simulink model "Ju_FCM_v2_03252019_Arash"  (R2018a)
settings: Solver=VariableStepAuto  StartTime=0.0  StopTime=.5  MaxStep=1e-6  RelTol=1e-3
values from neighbouring files (symbols this model uses):
  C_FCM = 100e-6    (= 0.0001)    [Ju_parameters_FCM_v2_03252019_Arash.m]
  f = 50    [Ju_parameters_FCM_v2_03252019_Arash.m]
  L = XL/(2*pi*f)    [Ju_parameters_FCM_v2_03252019_Arash.m]
  n = 4    [Ju_parameters_FCM_v2_03252019_Arash.m]
  R = Z*pf    (= 20)    [Ju_parameters_FCM_v2_03252019_Arash.m]
libraries: powerlib x21, powerlib_meascontrol x4
settings Model: Creator=JHK5183  LastModifiedBy=kzs1012
settings SolverCC: ZeroCrossAlgorithm=Adaptive
settings DebuggingCC: MaxConsecutiveZCsMsg=none

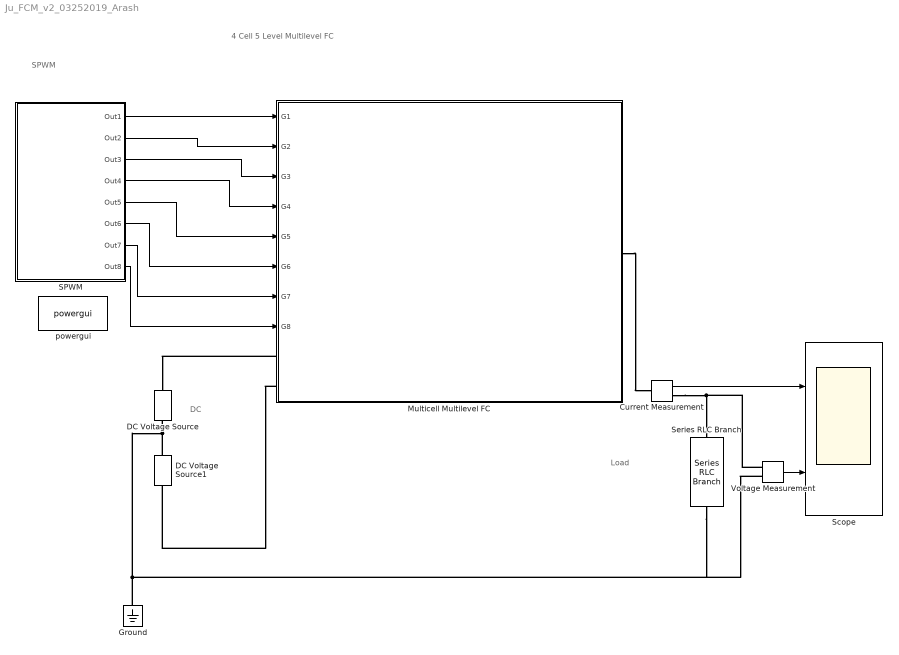
== system Ju_FCM_v2_03252019_Arash ==
  note: Load
  note: DC
  note: 4 Cell 5 Level Multilevel FC
  note: SPWM
  Current Measurement : powerlib/Measurements/Current Measurement  PhasorSimulation=off  OutputType=Complex  PSBequivalent=0
  DC Voltage Source : powerlib/Electrical Sources/DC Voltage Source  Amplitude=E/2  Measurements=None
  DC Voltage Source1 : powerlib/Electrical Sources/DC Voltage Source  Amplitude=E/2  Measurements=None
  Ground : powerlib/Elements/Ground  LConnTagsString=a
  Multicell Multilevel FC : Subsystem
  SPWM : Subsystem
  Scope : Scope  NumInputPorts=2
  Series RLC Branch : powerlib/Elements/Series RLC Branch  LConnTagsString=__new0  RConnTagsString=__new0  BranchType=RL  Resistance=R  Inductance=L  SetiL0=off  InitialCurrent=0  Capacitance=1e-6  Setx0=off  InitialVoltage=0  Measurements=None
  Voltage Measurement : powerlib/Measurements/Voltage Measurement  PhasorSimulation=off  OutputType=Complex  PSBequivalent=0
  powergui : powerlib/powergui  Priority=1  SimulationMode=Continuous  SampleTime=50e-6  frequency=60  Iterations=50  frequencyindice=0  Pbase=100e6  ErrMax=1e-4  UnitsV=kV  UnitsW=MW  buscounter=0  FunctionMessages=off  echomessages=off  EnableUseOfTLC=off  CurrentSourceSwitches=off  DisableSnubberDevices=off  DisableRonSwitches=off  DisableVfSwitches=off  DisplayEquations=off  SolverType=Tustin/Backward Euler (TBE)  Interpol=off  ExternalGateDelay=off  methode=off  Ts=100  x0status=blocks  SPID=on  SwTol=0  HookPort=off  RestoreLinks=warning  ResistiveCurrentMeasurement=off  Frange=[0:2:500]  Ylog=off  Xlog=on  ShowGrid=off  save=off  variable=ZData  structure=0  ZoomFFT=off  StartTime=0.0  cycles=1  DisplayStyle=1  fundamental=60  FreqAxis=off  MaxFrequency=1000  frequencyindicesteady=1  RmsSteady=1  display=off
  wires:
  Current Measurement/1 -> Scope/1
  Voltage Measurement/1 -> Scope/2
  SPWM/1(Out1) -> Multicell Multilevel FC/1(G1)
  SPWM/2(Out2) -> Multicell Multilevel FC/2(G2)
  SPWM/3(Out3) -> Multicell Multilevel FC/3(G3)
  SPWM/4(Out4) -> Multicell Multilevel FC/4(G4)
  SPWM/5(Out5) -> Multicell Multilevel FC/5(G5)
  SPWM/6(Out6) -> Multicell Multilevel FC/6(G6)
  SPWM/7(Out7) -> Multicell Multilevel FC/7(G7)
  SPWM/8(Out8) -> Multicell Multilevel FC/8(G8)
  connections:
  Multicell Multilevel FC/LConn1 -- DC Voltage Source/RConn1
  Voltage Measurement/LConn1 -- Current Measurement/RConn1 -- Series RLC Branch/LConn1
  DC Voltage Source/LConn1 -- Series RLC Branch/RConn1 -- Voltage Measurement/LConn2 -- Ground/LConn1 -- DC Voltage Source1/RConn1
  Multicell Multilevel FC/LConn2 -- DC Voltage Source1/LConn1
  Multicell Multilevel FC/RConn1 -- Current Measurement/LConn1

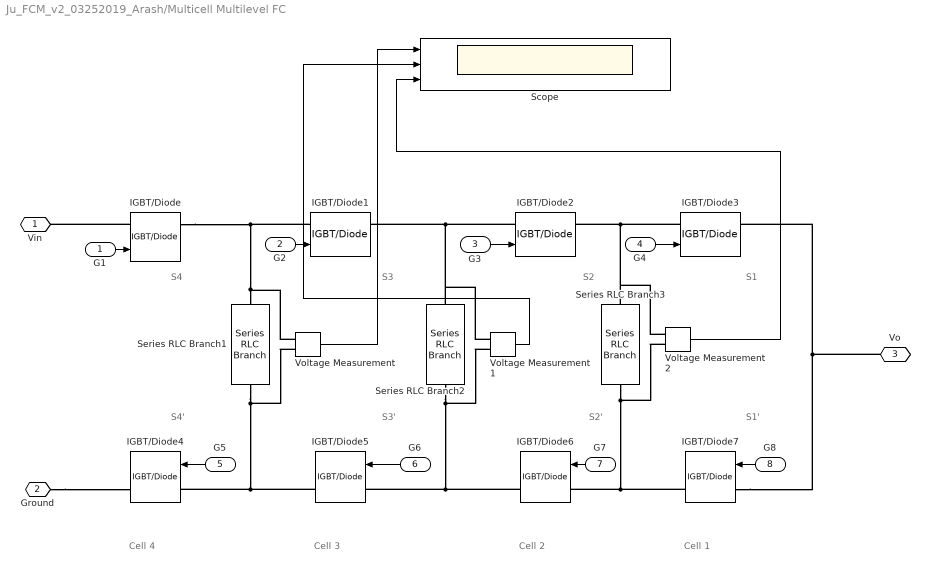
== system Ju_FCM_v2_03252019_Arash/Multicell Multilevel FC ==
  note: Cell 4
  note: S4
  note: S3
  note: S2
  note: S1
  note: S4'
  note: S3'
  note: S2'
  note: S1'
  note: Cell 3
  note: Cell 2
  note: Cell 1
  G1 : Inport
  G2 : Inport  Port=2
  G3 : Inport  Port=3
  G4 : Inport  Port=4
  G5 : Inport  Port=5
  G6 : Inport  Port=6
  G7 : Inport  Port=7
  G8 : Inport  Port=8
  IGBT/Diode{,1..7} (8 alike) : powerlib/Power Electronics/IGBT//Diode  Ron=1e-3  Rs=1e5  Cs=inf  Measurements=on
  Scope : Scope  NumInputPorts=3
  Series RLC Branch1 : powerlib/Elements/Series RLC Branch  LConnTagsString=__new0  RConnTagsString=__new0  BranchType=C  Resistance=1  Inductance=1e-3  SetiL0=off  InitialCurrent=0  Capacitance=C_FCM  Setx0=on  InitialVoltage=0  Measurements=None
  Series RLC Branch2 : powerlib/Elements/Series RLC Branch  LConnTagsString=__new0  RConnTagsString=__new0  BranchType=C  Resistance=1  Inductance=1e-3  SetiL0=off  InitialCurrent=0  Capacitance=C_FCM  Setx0=on  InitialVoltage=0  Measurements=None
  Series RLC Branch3 : powerlib/Elements/Series RLC Branch  LConnTagsString=__new0  RConnTagsString=__new0  BranchType=C  Resistance=1  Inductance=1e-3  SetiL0=off  InitialCurrent=0  Capacitance=C_FCM  Setx0=on  InitialVoltage=0  Measurements=None
  Voltage Measurement : powerlib/Measurements/Voltage Measurement  PhasorSimulation=off  OutputType=Complex  PSBequivalent=0
  Voltage Measurement1 : powerlib/Measurements/Voltage Measurement  PhasorSimulation=off  OutputType=Complex  PSBequivalent=0
  Voltage Measurement2 : powerlib/Measurements/Voltage Measurement  PhasorSimulation=off  OutputType=Complex  PSBequivalent=0
  Vin : PMIOPort  Side=Left
  Ground : PMIOPort  Port=2  Side=Left
  Vo : PMIOPort  Port=3  Side=Right
  wires:
  G1/1 -> IGBT/Diode/1
  G6/1 -> IGBT/Diode5/1
  G2/1 -> IGBT/Diode1/1
  G3/1 -> IGBT/Diode2/1
  G4/1 -> IGBT/Diode3/1
  G5/1 -> IGBT/Diode4/1
  G7/1 -> IGBT/Diode6/1
  G8/1 -> IGBT/Diode7/1
  Voltage Measurement/1 -> Scope/1
  Voltage Measurement1/1 -> Scope/2
  Voltage Measurement2/1 -> Scope/3
  connections:
  IGBT/Diode7/LConn1 -- IGBT/Diode3/RConn1 -- Vo/RConn1
  IGBT/Diode/RConn1 -- IGBT/Diode1/LConn1 -- Voltage Measurement/LConn1 -- Series RLC Branch1/LConn1
  IGBT/Diode/LConn1 -- Vin/RConn1
  IGBT/Diode2/LConn1 -- Voltage Measurement1/LConn1 -- Series RLC Branch2/LConn1 -- IGBT/Diode1/RConn1
  IGBT/Diode3/LConn1 -- Voltage Measurement2/LConn1 -- Series RLC Branch3/LConn1 -- IGBT/Diode2/RConn1
  Ground/RConn1 -- IGBT/Diode4/RConn1
  Series RLC Branch1/RConn1 -- Voltage Measurement/LConn2 -- IGBT/Diode4/LConn1 -- IGBT/Diode5/RConn1
  Series RLC Branch2/RConn1 -- Voltage Measurement1/LConn2 -- IGBT/Diode5/LConn1 -- IGBT/Diode6/RConn1
  Series RLC Branch3/RConn1 -- Voltage Measurement2/LConn2 -- IGBT/Diode6/LConn1 -- IGBT/Diode7/RConn1

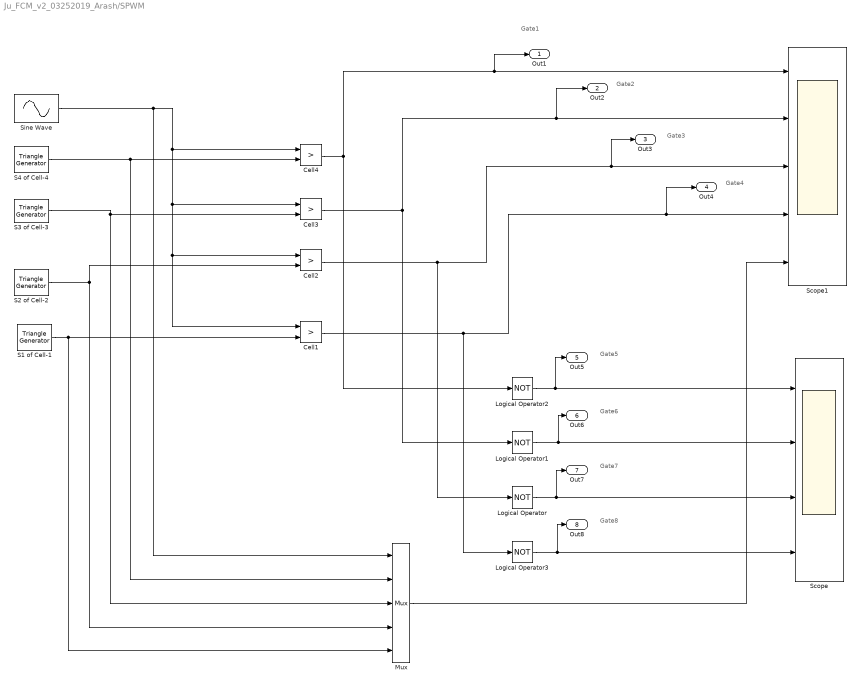
== system Ju_FCM_v2_03252019_Arash/SPWM ==
  note: Gate1
  note: Gate2
  note: Gate3
  note: Gate4
  note: Gate5
  note: Gate6
  note: Gate7
  note: Gate8
  Cell1 : RelationalOperator  Operator=>  OutDataTypeStr=boolean  RndMeth=Simplest
  Cell2 : RelationalOperator  Operator=>  OutDataTypeStr=boolean  RndMeth=Simplest
  Cell3 : RelationalOperator  Operator=>  OutDataTypeStr=boolean  RndMeth=Simplest
  Cell4 : RelationalOperator  Operator=>  OutDataTypeStr=boolean  ZeroCross=off  RndMeth=Simplest
  Logical Operator{,1..3} (4 alike) : Logic  Operator=NOT  AllPortsSameDT=off  OutDataTypeStr=boolean
  Mux : Mux  Inputs=5
  S1 of Cell-1 : powerlib_meascontrol/Pulse & Signal Generators/Triangle Generator  Freq=F_switch  Phase=0  Ts=0
  S2 of Cell-2 : powerlib_meascontrol/Pulse & Signal Generators/Triangle Generator  Freq=F_switch  Phase=360/n*3  Ts=0
  S3 of Cell-3 : powerlib_meascontrol/Pulse & Signal Generators/Triangle Generator  Freq=F_switch  Phase=360/n*2  Ts=0
  S4 of Cell-4 : powerlib_meascontrol/Pulse & Signal Generators/Triangle Generator  Freq=F_switch  Phase=360/n  Ts=0
  Scope : Scope  NumInputPorts=4
  Scope1 : Scope  NumInputPorts=5
  Sine Wave : Sin  Amplitude=.8  Frequency=2*pi*f  SampleTime=0  VectorParams1D=off
  Out1 : Outport
  Out2 : Outport  Port=2
  Out3 : Outport  Port=3
  Out4 : Outport  Port=4
  Out5 : Outport  Port=5
  Out6 : Outport  Port=6
  Out7 : Outport  Port=7
  Out8 : Outport  Port=8
  wires:
  Sine Wave/1 -> Mux/1, Cell4/1, Cell3/1, Cell2/1, Cell1/1
  S4 of Cell-4/1 -> Mux/2, Cell4/2
  S3 of Cell-3/1 -> Mux/3, Cell3/2
  S2 of Cell-2/1 -> Cell2/2, Mux/4
  S1 of Cell-1/1 -> Mux/5, Cell1/2
  Logical Operator2/1 -> Out5/1, Scope/1
  Logical Operator1/1 -> Out6/1, Scope/2
  Logical Operator/1 -> Out7/1, Scope/3
  Logical Operator3/1 -> Scope/4, Out8/1
  Mux/1 -> Scope1/5
  Cell4/1 -> Scope1/1, Out1/1, Logical Operator2/1
  Cell2/1 -> Logical Operator/1, Scope1/3, Out3/1
  Cell1/1 -> Logical Operator3/1, Scope1/4, Out4/1
  Cell3/1 -> Scope1/2, Out2/1, Logical Operator1/1
